simulink model "FINAL_MODEL_DOB"  (R2016a)
settings: Solver=VariableStepAuto  StartTime=0.0  StopTime=10  RelTol=1e-3
settings Model: Creator=Harsh Mathur  LastModifiedBy=Harsh Mathur

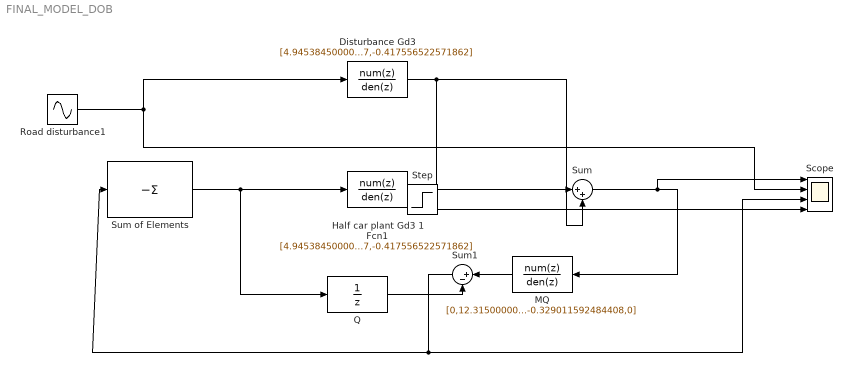
== system FINAL_MODEL_DOB ==
  Disturbance Gd3 : DiscreteTransferFcn  Numerator=[4.94538450000000,-16.1683393901000,18.4303307060006,-4.70382080898259,-7.34470352831246,6.39427693565206,-1.52013433786902,-0.0267173863676967]  Denominator=[1,-5.56300000000000,13.6494619999999,-19.2307473399999,16.8548157574011,-9.21660527305870,2.92363137823167,-0.417556522571862]  SampleTime=0.01  StateIdentifier=Gd1
  Half car plant Gd3 1 Fcn1 : DiscreteTransferFcn  Numerator=[4.94538450000000,-16.1683393901000,18.4303307060006,-4.70382080898259,-7.34470352831246,6.39427693565206,-1.52013433786902,-0.0267173863676967]  Denominator=[1,-5.56300000000000,13.6494619999999,-19.2307473399999,16.8548157574011,-9.21660527305870,2.92363137823167,-0.417556522571862]  SampleTime=0.01
  MQ : DiscreteTransferFcn  Numerator=[0,12.3150000000000,-68.5083450000000,168.093124530000,-236.826653492100,207.567056052381,-113.502493937734,36.0045204229271,-5.14220857547418]  Denominator=[60.9000000000000,-199.105220000000,226.960540681000,-57.9252608704228,-90.4464445331275,78.7424042319085,-18.7197135381940,-0.329011592484408,0]  SampleTime=0.01
  Q : DiscreteTransferFcn  Numerator=[0,1]  Denominator=[1,0]  SampleTime=0.01
  Road disturbance1 : Sin  SampleTime=0
  Scope : Scope  NumInputPorts=4
  Step : Step  SampleTime=0
  Sum : Sum  Inputs=|++
  Sum of Elements : Sum  Inputs=-
  Sum1 : Sum  Inputs=|+-
  wires:
  Road disturbance1/1 -> Scope/2, Disturbance Gd3/1
  Half car plant Gd3 1 Fcn1/1 -> Sum/1
  Q/1 -> Sum1/2
  Sum of Elements/1 -> Q/1, Half car plant Gd3 1 Fcn1/1
  Disturbance Gd3/1 -> Scope/4, Sum/2
  Sum1/1 -> Sum of Elements/1, Scope/3
  MQ/1 -> Sum1/1
  Sum/1 -> Scope/1, MQ/1
